simulink model "rudder_response"  (Simulink 6.6)
settings: Solver=ode3  StartTime=0.0  StopTime=3  FixedStep=T_step  RelTol=1e-3
values from neighbouring files (symbols this model uses):
  proportional_band = .5    (= 0.5)    [boat_constants.m]
  rudder_angle_dot_max = 10    [boat_constants.m]
  rudder_angle_max = 1    [boat_constants.m]
settings Model: Creator=Administrator  LastModifiedBy=Administrator

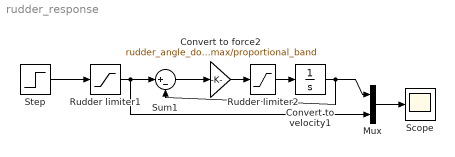
== system rudder_response ==
  Convert to force2 : Gain  Gain=rudder_angle_dot_max/proportional_band
  Convert to velocity1 : Integrator  LimitOutput=on  UpperSaturationLimit=rudder_angle_max  LowerSaturationLimit=-rudder_angle_max
  Mux : Mux  Inputs=2
  Rudder limiter1 : Saturate  UpperLimit=rudder_angle_max  LowerLimit=-rudder_angle_max
  Rudder limiter2 : Saturate  UpperLimit=rudder_angle_dot_max  LowerLimit=-rudder_angle_dot_max
  Scope : Scope
      settings: YMin=-1  YMax=2
  Step : Step  Before=1  After=0
  Sum1 : Sum  Inputs=|+-
  wires:
  Step/1 -> Rudder limiter1/1
  Convert to velocity1/1 -> Sum1/2, Mux/1
  Sum1/1 -> Convert to force2/1
  Rudder limiter1/1 -> Sum1/1, Mux/2
  Convert to force2/1 -> Rudder limiter2/1
  Mux/1 -> Scope/1
  Rudder limiter2/1 -> Convert to velocity1/1
